simulink model "TD_test"  (R2022b)
settings: Solver=FixedStepAuto  StartTime=0.0  StopTime=10  FixedStep=0.01  RelTol=1e-3
model workspace (MAT data in the model file):
  h = 0.01
  h0 = 0.01
  r0 = 1
settings Model: Creator=12854  LastModifiedBy=12854

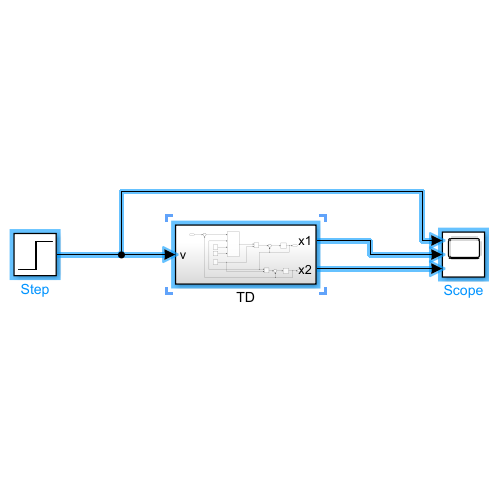
[thumbnail: Simulink's stored preview of the top-level diagram]
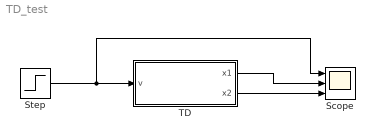
== system TD_test ==
  Scope : Scope  NumInputPorts=3
  Step : Step  SampleTime=0
  TD : Subsystem
  wires:
  TD/1(x1) -> Scope/2
  TD/2(x2) -> Scope/3
  Step/1 -> Scope/1, TD/1(v)

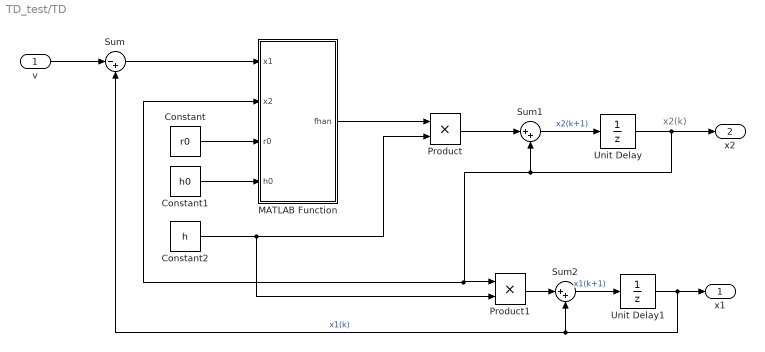
== system TD_test/TD ==
  note: x2(k)
  v : Inport
  Constant : Constant  Value=r0
  Constant1 : Constant  Value=h0
  Constant2 : Constant  Value=h
  MATLAB Function : MATLAB Function  TreatAsAtomicUnit=on
  Product : Product
  Product1 : Product
  Sum : Sum  Inputs=|-+
  Sum1 : Sum  Inputs=|++
  Sum2 : Sum  Inputs=|++
  Unit Delay : UnitDelay  SampleTime=-1  HasFrameUpgradeWarning=on
  Unit Delay1 : UnitDelay  SampleTime=-1  HasFrameUpgradeWarning=on
  x1 : Outport
  x2 : Outport  Port=2
  wires:
  Product1/1 -> Sum2/1
  Unit Delay1/1 -> Sum2/2, Sum/2, x1/1  "x1(k)"
  Sum1/1 -> Unit Delay/1  "x2(k+1)"
  Sum/1 -> MATLAB Function/1(x1)
  Constant/1 -> MATLAB Function/3(r0)
  Constant1/1 -> MATLAB Function/4(h0)
  MATLAB Function/1(fhan) -> Product/1
  v/1 -> Sum/1
  Constant2/1 -> Product1/2, Product/2
  Product/1 -> Sum1/1
  Sum2/1 -> Unit Delay1/1  "x1(k+1)"
  Unit Delay/1 -> Product1/1, MATLAB Function/2(x2), Sum1/2, x2/1

== matlab function TD_test/TD/MATLAB Function ==
  data: x1 input; fhan output; x2 input; r0 input; h0 input
% ADRC中的fhan函数（最速综合函数，TD、NLSEF使用）
function fhan = fhan(x1,x2,r0,h0)
d = r0 * (h0^2);
a0 = h0 * x2;
y = x1 + a0;
a1 = sqrt(d * (d + 8 * abs(y)));
a2 = a0 + sign(y) * (a1 - d)/2;
sy = (sign(y + d) - sign(y - d))/2;
a = (a0 + y - a2) * sy + a2;
sa = (sign(a + d) - sign(a - d))/2;
fhan = -r0 * (a / d - sign(a)) * sa - r0 * sign(a);
